simulink model "KakmanFilterSensorFusion__Simtestbench"  (R2023b)
settings: Solver=FixedStepAuto  StartTime=0.0  StopTime=tend  FixedStep=Ts  RelTol=1e-3
undefined symbols (not defined in the file): Discrete, Time, Ts
libraries: ctrlSharedLib x2
settings Model: Creator=leoni  LastModifiedBy=leoni

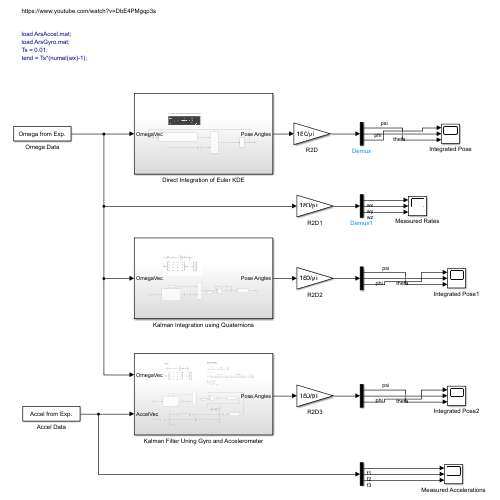
[thumbnail: Simulink's stored preview of the top-level diagram]
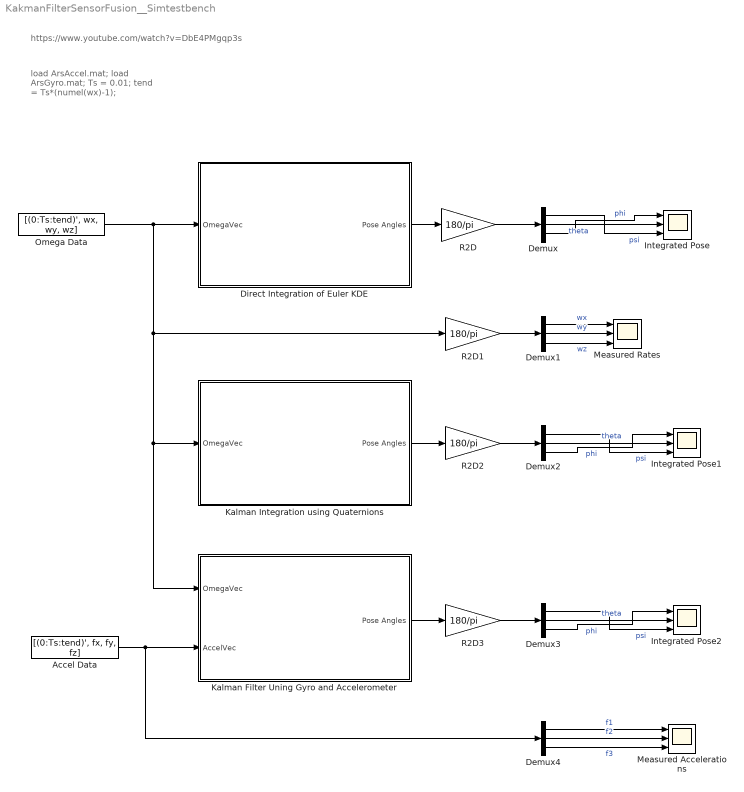
== system KakmanFilterSensorFusion__Simtestbench ==
  note: https://www.youtube.com/watch?v=DbE4PMgqp3s
  note: load ArsAccel.mat;
      | load ArsGyro.mat;
      | Ts = 0.01;
      | tend = Ts*(numel(wx)-1);
  Accel Data : FromWorkspace  VariableName=[(0:Ts:tend)', fx, fy, fz]
      mask Display: disp('Accel from Exp.')
  Demux{,1..4} (5 alike) : Demux  Outputs=3
  Direct Integration of Euler KDE : Subsystem
  Integrated Pose : Scope  NumInputPorts=3
  Integrated Pose1 : Scope  NumInputPorts=3
  Integrated Pose2 : Scope  NumInputPorts=3
  Kalman Filter Uning Gyro and Accelerometer : Subsystem
  Kalman Integration using Quaternions : Subsystem
  Measured Accelerations : Scope  NumInputPorts=3
  Measured Rates : Scope  NumInputPorts=3
  Omega Data : FromWorkspace  VariableName=[(0:Ts:tend)', wx, wy, wz]
      mask Display: disp('Omega from Exp.')
  R2D{,1..3} (4 alike) : Gain  Gain=180/pi
  wires:
  Omega Data/1 -> R2D1/1, Kalman Filter Uning Gyro and Accelerometer/1(OmegaVec), Kalman Integration using Quaternions/1(OmegaVec), Direct Integration of Euler KDE/1(OmegaVec)
  Direct Integration of Euler KDE/1(Pose Angles) -> R2D/1
  Demux/1 -> Integrated Pose/3  "psi"
  Demux/2 -> Integrated Pose/2  "theta"
  Demux/3 -> Integrated Pose/1  "phi"
  Demux1/1 -> Measured Rates/1  "wx"
  Demux1/2 -> Measured Rates/2  "wy"
  Demux1/3 -> Measured Rates/3  "wz"
  R2D/1 -> Demux/1
  R2D1/1 -> Demux1/1
  Kalman Integration using Quaternions/1(Pose Angles) -> R2D2/1
  R2D2/1 -> Demux2/1
  Demux2/3 -> Integrated Pose1/1  "phi"
  Demux2/2 -> Integrated Pose1/2  "theta"
  Demux2/1 -> Integrated Pose1/3  "psi"
  Accel Data/1 -> Demux4/1, Kalman Filter Uning Gyro and Accelerometer/2(AccelVec)
  Demux3/1 -> Integrated Pose2/3  "psi"
  Demux3/2 -> Integrated Pose2/2  "theta"
  Demux3/3 -> Integrated Pose2/1  "phi"
  R2D3/1 -> Demux3/1
  Kalman Filter Uning Gyro and Accelerometer/1(Pose Angles) -> R2D3/1
  Demux4/1 -> Measured Accelerations/1  "f1"
  Demux4/2 -> Measured Accelerations/2  "f2"
  Demux4/3 -> Measured Accelerations/3  "f3"

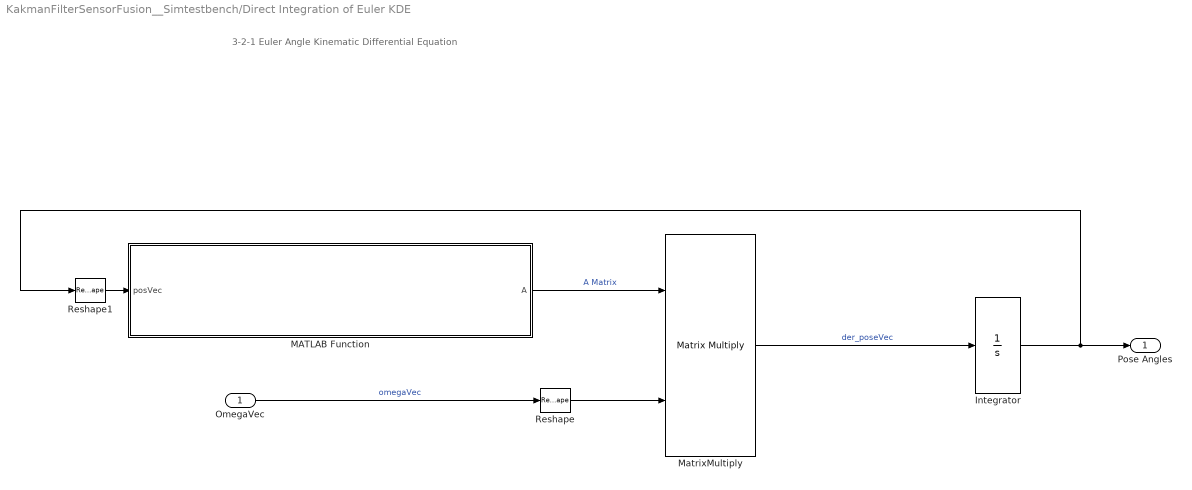
== system KakmanFilterSensorFusion__Simtestbench/Direct Integration of Euler KDE ==
  note: 3-2-1 Euler Angle Kinematic Differential Equation
  OmegaVec : Inport
  Integrator : Integrator  InitialCondition=[0;0;0]
  MATLAB Function : MATLAB Function  TreatAsAtomicUnit=on
  MatrixMultiply : Product  Multiplication=Matrix(*)
  Reshape : Reshape  OutputDimensionality=Column vector (2-D)
  Reshape1 : Reshape  OutputDimensionality=Column vector (2-D)
  Pose Angles : Outport
  wires:
  OmegaVec/1 -> Reshape/1  "omegaVec"
  MATLAB Function/1(A) -> MatrixMultiply/1  "A Matrix"
  MatrixMultiply/1 -> Integrator/1  "der_poseVec"
  Integrator/1 -> Reshape1/1, Pose Angles/1
  Reshape/1 -> MatrixMultiply/2
  Reshape1/1 -> MATLAB Function/1(posVec)

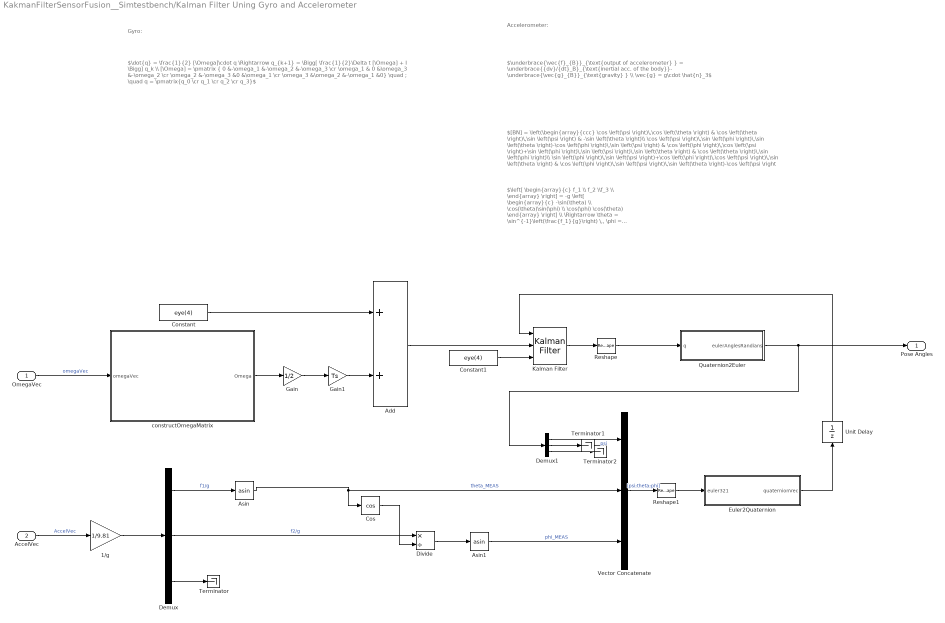
== system KakmanFilterSensorFusion__Simtestbench/Kalman Filter Uning Gyro and Accelerometer ==
  note: $\left[ \begin{array}{c} f_1 \\ f_2 \\f_3 \\ \end{array} \right] = -g \left[ \begin{array}{c} -\sin(\theta) \\ \cos(\theta)\sin(\phi) \\ \cos(\phi) \cos(\theta) \end{array} \right] \\ \Rightarrow \theta = \sin^{-1}\left(\frac{f_1}{g}\right) \,, \phi = \sin^{-1} \left(\frac{-f_2}{g \cos\theta}\right)$
  note: $[BN] = \left(\begin{array}{ccc} \cos \left(\psi \right)\,\cos \left(\theta \right) & \cos \left(\theta \right)\,\sin \left(\psi \right) & -\sin \left(\theta \right)\\ \cos \left(\psi \right)\,\sin \left(\phi \right)\,\sin \left(\theta \right)-\cos \left(\phi \right)\,\sin \left(\psi \right) & \cos \left(\phi \right)\,\cos \left(\psi \right)+\sin \left(\phi \right)\,\sin \left(\psi \right)\,\sin \left(\theta \right) & \cos \left(\theta \right)\,\sin \left(\phi \right)\\ \sin \left(\phi \right)\,\sin \left(\psi \right)+\cos \left(\phi \right)\,\cos \left(\psi \right)\,\sin \left(\theta \right) & \cos \left(\phi \right)\,\sin \left(\psi \right)\,\sin \left(\theta \right)-\cos \left(\psi \right)\,\sin \left(\phi \right) & \cos \left(\phi \right)\,\cos \left(\theta \right) \end{array}\right)$
  note: $\underbrace{\vec{f}_{B}}_{\text{output of accelerometer} } = \underbrace{{dv}/{dt}_B}_{\text{inertial acc. of the body}}- \underbrace{\vec{g}_{B}}_{\text{gravity} } \\ \vec{g} = g\cdot \hat{n}_3$
  note: Gyro:
  note: $\dot{q} = \frac{1}{2} [\Omega]\cdot q \Rightarrow q_{k+1} = \Bigg[ \frac{1}{2}\Delta t [\Omega] + I \Bigg] q_k \\ [\Omega] = \pmatrix { 0 &-\omega_1 &-\omega_2 &-\omega_3 \cr \omega_1 & 0 &\omega_3 &-\omega_2 \cr \omega_2 &-\omega_3 &0 &\omega_1 \cr \omega_3 &\omega_2 &-\omega_1 &0} \quad ; \quad q = \pmatrix{q_0 \cr q_1 \cr q_2 \cr q_3}$
  note: Accelerometer:
  OmegaVec : Inport  SampleTime=Ts
  AccelVec : Inport  Port=2  SampleTime=Ts
  1/g : Gain  Gain=1/9.81
  Add : Sum
  Asin : Trigonometry  Operator=asin
  Asin1 : Trigonometry  Operator=asin
  Constant : Constant  Value=eye(4)  SampleTime=Ts
  Constant1 : Constant  Value=eye(4)  SampleTime=Ts
  Cos : Trigonometry  Operator=cos
  Demux : Demux  Outputs=3
  Demux1 : Demux  Outputs=3
  Divide : Product  Inputs=*/
  Euler2Quaternion : MATLAB Function  TreatAsAtomicUnit=on
  Gain : Gain  Gain=1/2
  Gain1 : Gain  Gain=Ts
  Kalman Filter : ctrlSharedLib/Kalman Filter  TimeDomain=Discrete-Time  UseCurrentEstimator=on  ModelSource=Input port  ModelSourceVariable=ss(0.95,1,1,0,1)  A=0.95  B=1  C=1  D=0  NumberOfStates=4  NumberOfInputs=1  NumberOfOutputs=4  InitialEstimateSource=Dialog  X0=[1;0;0;0]  P0=eye(4)  UseK=off  UseGH=off  NumberOfProcessNoiseInputs=1  G=1  TimeInvariantG=on  H=0  TimeInvariantH=on  Q=0.0001*eye(4)  TimeInvariantQ=on  R=10*eye(4)  TimeInvariantR=on  N=0  TimeInvariantN=on  AddInputPort=off  AddEnablePort=off  OutputEstimatedY=off  OutputP=off  Ts=Ts
  Quaternion2Euler : MATLAB Function  TreatAsAtomicUnit=on
  Reshape : Reshape  OutputDimensionality=Column vector (2-D)
  Reshape1 : Reshape  OutputDimensionality=Row vector (2-D)
  Terminator : Terminator
  Terminator1 : Terminator
  Terminator2 : Terminator
  Unit Delay : UnitDelay  SampleTime=-1  HasFrameUpgradeWarning=on
  Vector Concatenate : Concatenate  NumInputs=3
  constructOmegaMatrix : MATLAB Function  TreatAsAtomicUnit=on
  Pose Angles : Outport
  wires:
  Reshape/1 -> Quaternion2Euler/1(q)
  Constant1/1 -> Kalman Filter/3
  Add/1 -> Kalman Filter/2
  Constant/1 -> Add/1
  Gain/1 -> Gain1/1
  Gain1/1 -> Add/2
  Kalman Filter/1 -> Reshape/1
  constructOmegaMatrix/1(Omega) -> Gain/1
  OmegaVec/1 -> constructOmegaMatrix/1(omegaVec)  "omegaVec"
  AccelVec/1 -> 1/g/1  "AccelVec"
  Demux/1 -> Asin/1  "f1/g"
  Demux/2 -> Divide/1  "f2/g"
  1/g/1 -> Demux/1
  Demux/3 -> Terminator/1
  Asin/1 -> Cos/1, Vector Concatenate/2  "theta_MEAS"
  Cos/1 -> Divide/2
  Divide/1 -> Asin1/1
  Asin1/1 -> Vector Concatenate/3  "phi_MEAS"
  Vector Concatenate/1 -> Reshape1/1  "[psi;theta;phi]"
  Demux1/2 -> Terminator1/1
  Demux1/3 -> Terminator2/1
  Demux1/1 -> Vector Concatenate/1  "psi"
  Euler2Quaternion/1(quaternionVec) -> Unit Delay/1
  Unit Delay/1 -> Kalman Filter/1
  Quaternion2Euler/1(eulerAnglesRandians) -> Demux1/1, Pose Angles/1
  Reshape1/1 -> Euler2Quaternion/1(euler321)

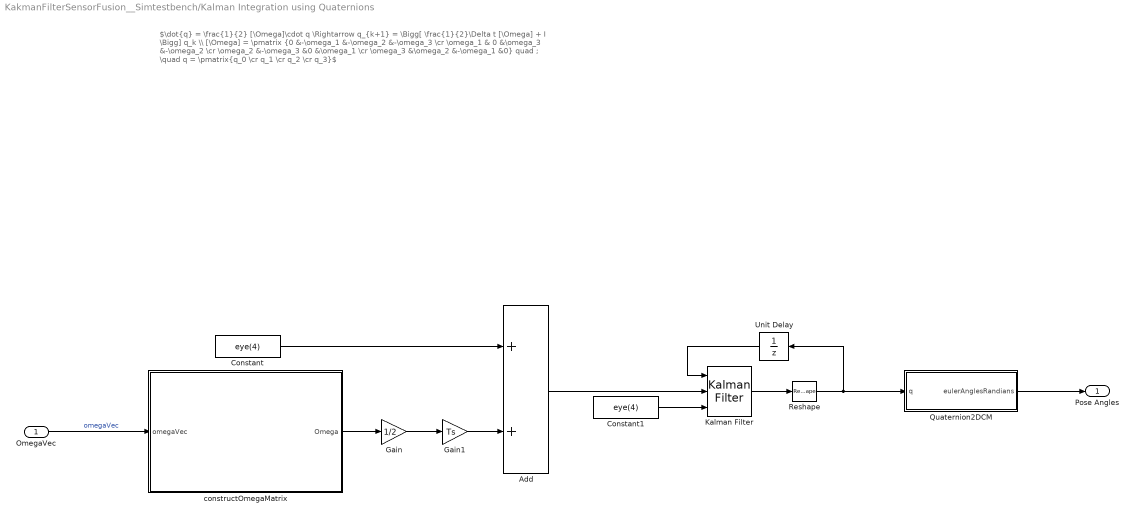
== system KakmanFilterSensorFusion__Simtestbench/Kalman Integration using Quaternions ==
  note: $\dot{q} = \frac{1}{2} [\Omega]\cdot q \Rightarrow q_{k+1} = \Bigg[ \frac{1}{2}\Delta t [\Omega] + I \Bigg] q_k \\ [\Omega] = \pmatrix {0 &-\omega_1 &-\omega_2 &-\omega_3 \cr \omega_1 & 0 &\omega_3 &-\omega_2 \cr \omega_2 &-\omega_3 &0 &\omega_1 \cr \omega_3 &\omega_2 &-\omega_1 &0} quad ; \quad q = \pmatrix{q_0 \cr q_1 \cr q_2 \cr q_3}$
  OmegaVec : Inport  SampleTime=Ts
  Add : Sum
  Constant : Constant  Value=eye(4)  SampleTime=Ts
  Constant1 : Constant  Value=eye(4)  SampleTime=Ts
  Gain : Gain  Gain=1/2
  Gain1 : Gain  Gain=Ts
  Kalman Filter : ctrlSharedLib/Kalman Filter  TimeDomain=Discrete-Time  UseCurrentEstimator=on  ModelSource=Input port  ModelSourceVariable=ss(0.95,1,1,0,1)  A=0.95  B=1  C=1  D=0  NumberOfStates=4  NumberOfInputs=1  NumberOfOutputs=4  InitialEstimateSource=Dialog  X0=[1;0;0;0]  P0=eye(4)  UseK=off  UseGH=off  NumberOfProcessNoiseInputs=1  G=1  TimeInvariantG=on  H=0  TimeInvariantH=on  Q=0.0001*eye(4)  TimeInvariantQ=on  R=10*eye(4)  TimeInvariantR=on  N=0  TimeInvariantN=on  AddInputPort=off  AddEnablePort=off  OutputEstimatedY=off  OutputP=off  Ts=Ts
  Quaternion2DCM : MATLAB Function  TreatAsAtomicUnit=on
  Reshape : Reshape  OutputDimensionality=Column vector (2-D)
  Unit Delay : UnitDelay  SampleTime=-1  HasFrameUpgradeWarning=on
  constructOmegaMatrix : MATLAB Function  TreatAsAtomicUnit=on
  Pose Angles : Outport
  wires:
  OmegaVec/1 -> constructOmegaMatrix/1(omegaVec)  "omegaVec"
  constructOmegaMatrix/1(Omega) -> Gain/1
  Kalman Filter/1 -> Reshape/1
  Gain1/1 -> Add/2
  Gain/1 -> Gain1/1
  Constant/1 -> Add/1
  Add/1 -> Kalman Filter/2
  Constant1/1 -> Kalman Filter/3
  Quaternion2DCM/1(eulerAnglesRandians) -> Pose Angles/1
  Reshape/1 -> Quaternion2DCM/1(q), Unit Delay/1
  Unit Delay/1 -> Kalman Filter/1

== matlab function KakmanFilterSensorFusion__Simtestbench/Direct Integration of Euler KDE/MATLAB Function ==
  data: posVec input; A output
function  A = fcn(posVec)

phi = posVec(3);
theta = posVec(2);
psi = posVec(1);


MAT = [    0              sin(phi)                cos(phi);...
         0          cos(phi)*cos(theta)     -sin(phi)*cos(theta);...
     cos(theta)    sin(phi)*sin(theta)      cos(phi)*sin(theta)];


A =1/cos(theta)*MAT;
end

== matlab function KakmanFilterSensorFusion__Simtestbench/Kalman Integration using Quaternions/Quaternion2DCM ==
  data: q input; eulerAnglesRandians output
function eulerAnglesRandians = fcn(q)
quat = quaternion([q(1) q(2) q(3) q(4)]);

eulerAnglesRandians = euler(quat,"ZYX","frame");

end

== matlab function KakmanFilterSensorFusion__Simtestbench/Kalman Filter Uning Gyro and Accelerometer/Quaternion2Euler ==
  data: q input; eulerAnglesRandians output
function eulerAnglesRandians = fcn(q)

quat = quaternion([q(1) q(2) q(3) q(4)]);

eulerAnglesRandians = euler(quat,"ZYX","frame");

end

== matlab function KakmanFilterSensorFusion__Simtestbench/Kalman Filter Uning Gyro and Accelerometer/constructOmegaMatrix ==
  data: omegaVec input; Omega output
function  Omega = fcn(omegaVec)

w1 = omegaVec(1);
w2 = omegaVec(2);
w3 = omegaVec(3);


Omega = [0 -w1 -w2 -w3;...
         w1 0   w3 -w2;...
         w2 -w3 0 w1;...
         w3 w2 -w1 0];

== matlab function KakmanFilterSensorFusion__Simtestbench/Kalman Filter Uning Gyro and Accelerometer/Euler2Quaternion ==
  data: euler321 input; quaternionVec output
function quaternionVec = fcn(euler321)


quaternionVec =  compact(quaternion(euler321,"euler","ZYX","frame"));

end

== matlab function KakmanFilterSensorFusion__Simtestbench/Kalman Integration using Quaternions/constructOmegaMatrix ==
  data: omegaVec input; Omega output
function  Omega = fcn(omegaVec)

w1 = omegaVec(1);
w2 = omegaVec(2);
w3 = omegaVec(3);


Omega = [0 -w1 -w2 -w3;...
         w1 0   w3 -w2;...
         w2 -w3 0 w1;...
         w3 w2 -w1 0];
